simulink model "SphericalTanks"  (R2018a)
settings: Solver=ode45  StartTime=0.0  StopTime=200  RelTol=1e-6
values from neighbouring files (symbols this model uses):
  du = 0.1    [TanqueEsf.m]
  F1 = 1.75    [TanqueEsf.m]
  F2 = 1    [TanqueEsf.m]
  h1s = X(1)    [TanqueEsf.m]    (also in interac.m)
  h2s = X(2)    [TanqueEsf.m]    (also in interac.m)
undefined symbols (not defined in the file or in its folder): par
libraries: cstblocks x1
settings Model: Creator=Sergio  LastModifiedBy=Sergio
settings CodeAppCC: StateflowObjectComments=on

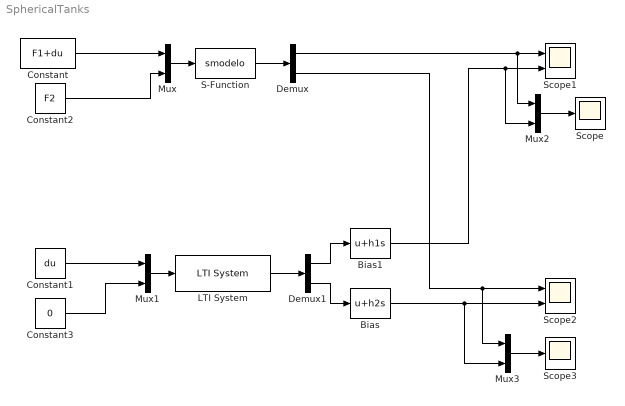
== system SphericalTanks ==
  Bias : Bias  Bias=h2s
  Bias1 : Bias  Bias=h1s
  Constant : Constant  Value=F1+du
  Constant1 : Constant  Value=du
  Constant2 : Constant  Value=F2
  Constant3 : Constant  Value=0
  Demux : Demux  Outputs=2
  Demux1 : Demux  Outputs=2
  LTI System : cstblocks/LTI System  sys=H  IC=[]
  Mux{,1..3} (4 alike) : Mux  Inputs=2
  S-Function : S-Function  FunctionName=smodelo  Parameters=par,h1s,h2s  SFunctionDeploymentMode=off  EnableBusSupport=off
  Scope : Scope
  Scope1 : Scope  NumInputPorts=2
  Scope2 : Scope  NumInputPorts=2
  Scope3 : Scope
  wires:
  Constant/1 -> Mux/1
  Constant2/1 -> Mux/2
  Mux/1 -> S-Function/1
  S-Function/1 -> Demux/1
  Mux1/1 -> LTI System/1
  Constant1/1 -> Mux1/1
  Constant3/1 -> Mux1/2
  LTI System/1 -> Demux1/1
  Demux1/2 -> Bias/1
  Demux1/1 -> Bias1/1
  Demux/1 -> Mux2/1, Scope1/1
  Bias1/1 -> Mux2/2, Scope1/2
  Bias/1 -> Mux3/2, Scope2/2
  Demux/2 -> Mux3/1, Scope2/1
  Mux2/1 -> Scope/1
  Mux3/1 -> Scope3/1
